simulink model "addsub"  (R2016a)
settings: Solver=FixedStepDiscrete  StartTime=0.0  StopTime=10.0  RelTol=1e-3
libraries: rvs x8
settings Model: Creator=Arthur  LastModifiedBy=arthur
settings DataIOCC: LimitDataPoints=on  SaveFormat=Array
settings DebuggingCC: SolverPrmCheckMsg=warning
settings HardwareCC: ProdBitPerPointer=32  ProdLargestAtomicFloat=None  ProdIntDivRoundTo=Undefined  ProdEndianess=Unspecified  ProdWordSize=32  ProdHWDeviceType=32-bit Generic
settings ModelReferenceCC: PropagateSignalLabelsOutOfModel=off
settings ConfigComp: CovModelRefEnable=Off  CovSFcnEnable=off

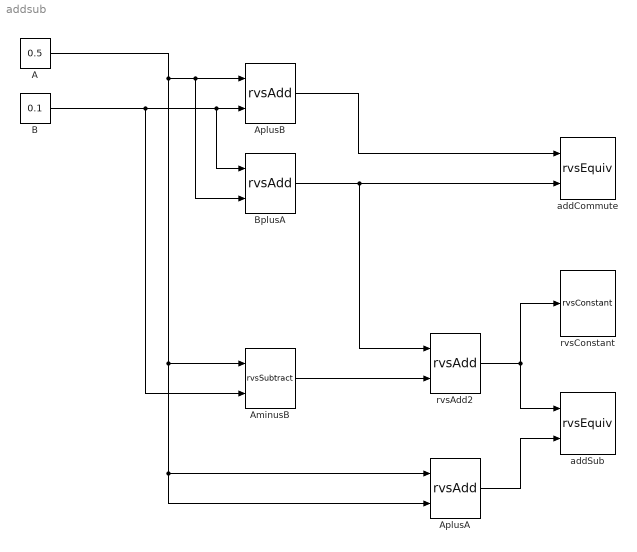
== system addsub ==
  A : Constant  Value=0.5
  AminusB : rvs/rvsSubtract
  AplusA : rvs/rvsAdd
  AplusB : rvs/rvsAdd
  B : Constant  Value=0.1
  BplusA : rvs/rvsAdd
  addCommute : rvs/rvsEquiv  tol=1e-9
  addSub : rvs/rvsEquiv  tol=1e-9
  rvsAdd2 : rvs/rvsAdd
  rvsConstant : rvs/rvsConstant
  wires:
  B/1 -> AminusB/2, BplusA/1, AplusB/2
  AplusB/1 -> addCommute/1
  AminusB/1 -> rvsAdd2/2
  BplusA/1 -> rvsAdd2/1, addCommute/2
  rvsAdd2/1 -> rvsConstant/1, addSub/1
  AplusA/1 -> addSub/2
  A/1 -> AplusA/2, AplusA/1, AminusB/1, BplusA/2, AplusB/1
